simulink model "PC_CONTROL_STATION"  (R2023b)
settings: Solver=FixedStepAuto  StartTime=0.0  StopTime=inf  RelTol=1e-3  EnableMultiTasking=on
InitFcn:
  | if RUN_MODE~=5
  |     % clear rpi;
  |     rpi = raspberrypi(CAR_IP, 'pi', 'LabControl');
  |     stopModel(rpi,'CAR_CONTROL_SYSTEM')
  |     while isModelRunning(rpi,'CAR_CONTROL_SYSTEM')
  |          stopModel(rpi,'CAR_CONTROL_SYSTEM')
  |     end
  |     runModel(rpi,'CAR_CONTROL_SYSTEM')
  |      while isModelRunning(rpi,'CAR_CONTROL_SYSTEM')==false
  |          runModel(rpi,'CAR_CONTROL_SYSTEM')
  |      end
  |      % clear rpi;
  | end
StopFcn:
  | if RUN_MODE~=5
  |    clear rpi;
  |    rpi = raspberrypi(CAR_IP, 'pi', 'LabControl');
  |    stopModel(rpi,'CAR_CONTROL_SYSTEM')
  |    while isModelRunning(rpi,'CAR_CONTROL_SYSTEM')
  |    end
  |    clear rpi;
  | end
model workspace (MAT data in the model file):
  SL_ROS_VariableLengthArrays_MaxSizes : object (value not decoded)
values from neighbouring files (symbols this model uses):
  data = theClient.GetLastFrameOfData()    [FuncMotive.m]
undefined symbols (not defined in the file or in its folder): CONTROL, CONTROL_INI, data_SL_Info, MD25, MSG, SAMPLING_TIME, Standard_Devices, SYSID_INPUT, TCP_Protocol, UDP_Protocol
libraries: simulink x51, sldrtlib x46, dspsigattribs x7, ros2lib x3, ctrlSharedLib x2, aerolibanimutils x1
(part 4 of 8)

== matlab function PC_CONTROL_STATION/PC TARGETS/PC TARGETS/YAW RATE TARGET/ PULSE GENERATION  ==
  data: CONTROL input Bus: CONTROL_Bus; YAW_RATE_REF output
function YAW_RATE_REF = PULSE_GEN(CONTROL)
    
persistent TIMER initialize
if isempty(initialize)
    TIMER = 0;
    initialize = 1;
end

% SAMPLING TIME
SAMPLING_TIME = CONTROL.PARAM.SAMPLING_TIME; % s

%% OPERATION MODE
% / 0. BOOTING   / 1. SENSOR CALIBRATION / 2. READY
% / 3. OPEN LOOP / 4. ATTITUDE / 5. VELOCITY / 6. NAVIGATION / 
% / 7. WALL FOLLOWER / 8. WALL-FOLLOWER COMPETITION / 
% / 9. NAVIGATION COMPETITION / 10. STOP
CURRENT_STATUS = CONTROL.STATE.CURRENT_STATUS_SYS;
PREVIOUS_STATUS = CONTROL.STATE.PREVIOUS_STATUS;

if (CURRENT_STATUS == 5) && (PREVIOUS_STATUS == 5)   
    if TIMER > 7.5
        YAW_RATE_REF = 0;
    elseif TIMER < 5
        YAW_RATE_REF = 0;
        TIMER = TIMER + SAMPLING_TIME;
    else % 5 <= TIMER <= 7.5
        YAW_RATE_REF = 30*pi/180;
        TIMER = TIMER + SAMPLING_TIME;
    end
else
    YAW_RATE_REF = 0;
    TIMER = 0;
end

== matlab function PC_CONTROL_STATION/PC TARGETS/PC TARGETS/FORWARD VELOCITY TARGET/RAMP ==
  data: SAMPLING_TIME input; ramp_out output
function ramp_out = RAMP(SAMPLING_TIME)

%--------------------------------------------------------------
% PERSISTENT VARIABLES
%--------------------------------------------------------------
persistent ramp ramp_slope TIMER initialize
if isempty(initialize)
    TIMER = 0;
    ramp = 1;
    ramp_slope = -1;
    initialize = 1;
end

TIMER = TIMER + SAMPLING_TIME;
if TIMER < 30
    ramp_out = ramp; 
    return
else
    TIMER = 0;
end

if ramp==1 || ramp==4
    ramp_slope = -ramp_slope;
end

ramp = ramp + ramp_slope;

ramp_out = ramp;
